simulink model "G2V"  (R2023b)
settings: Solver=VariableStepAuto  StartTime=0.0  StopTime=5  RelTol=1e-3
libraries: spsIGBTDiodeLib x4, spsSeriesRLCBranchLib x3, spsVoltageMeasurementLib x2, spsACVoltageSourceLib x1, spsDiodeLib x1, spsMosfetLib x1, slpidlib x1, spsPWMGeneratorDCDCLib x1, spsTriangleGeneratorLib x1, sps_lib x1
settings Model: Creator=armaan  LastModifiedBy=armaan

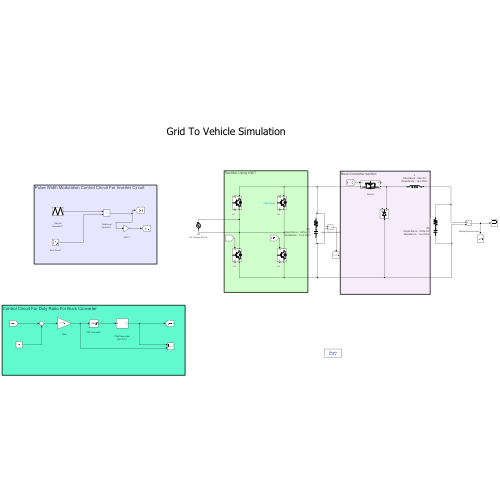
[thumbnail: Simulink's stored preview of the top-level diagram]
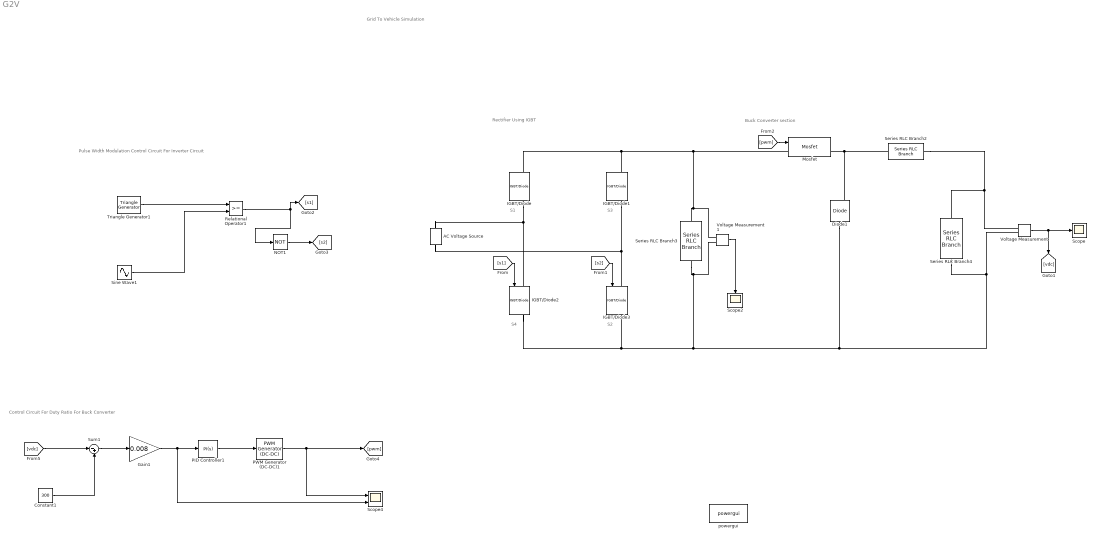
== system G2V ==
  note: Grid To Vehicle Simulation
  note: S1
  note: Buck Converter section
  note: Rectifier Using IGBT
  note: Pulse Width Modulation Control Circuit For Inverter Circuit
  note: Control Circuit For Duty Ratio For Buck Converter
  note: S3
  note: S2
  note: S4
  AC Voltage Source : spsACVoltageSourceLib/AC Voltage Source  Amplitude=440  Phase=0  Frequency=50  SampleTime=0  Measurements=None  BusType=swing  Pref=10e3  Qref=0  Qmin=-inf  Qmax=+inf
      settings: AttributesFormatString=|
      | %<Amplitude>
      | %<Name>
  Constant1 : Constant  Value=300
  Diode1 : spsDiodeLib/Diode  Ron=1e-3  Lon=0  Vf=0  IC=0  UseSnubber=off  Rs=inf  Cs=inf  Measurements=on
  Gain1 : Gain  Gain=0.008
      settings: AttributesFormatString=%<BlockType>
  IGBT/Diode{,1..3} (4 alike) : spsIGBTDiodeLib/IGBT//Diode  Ron=1e-3  Rs=1e5  Cs=inf  Measurements=on
  Mosfet : spsMosfetLib/Mosfet  Ron=0.1  Lon=0  Rd=0.01  Vfd=0  IC=0  Rs=1e5  Cs=inf  Measurements=on
      settings: AttributesFormatString=%<Name>
  NOT1 : Logic  Operator=NOT  IconShape=distinctive  AllPortsSameDT=off  OutDataTypeStr=boolean
      settings: AttributesFormatString=%<Name>
  PID Controller1 : slpidlib/PID Controller  Controller=PI  Form=Parallel  TimeDomain=Continuous-time  UseExternalTs=off  SampleTime=-1  IntegratorMethod=Forward Euler  FilterMethod=Forward Euler  ControllerParametersSource=internal  P=0.1  I=0.1  UseKiTs=off  D=0.1  N=100  UseFilter=on  TunerSelectOption=Transfer Function Based (PID Tuner App)  InitialConditionSource=internal  InitialConditionForIntegrator=0  InitialConditionForFilter=0  DifferentiatorICPrevScaledInput=0  ExternalReset=none  TrackingMode=off  Kt=1  LimitOutput=on  SatLimitsSource=internal  UpperSaturationLimit=1  LowerSaturationLimit=0  LinearizeAsGain=on  AntiWindupMode=none  Kb=1  LimitIntegrator=off  UpperIntegratorSaturationLimit=inf  LowerIntegratorSaturationLimit=-inf  POutMin=[]  POutMax=[]  IOutMin=[]  IOutMax=[]  DOutMin=[]  DOutMax=[]  NOutMin=[]  NOutMax=[]  SumOutMin=[]  SumOutMax=[]  SaturationOutMin=[]  SaturationOutMax=[]  PParamMin=[]  PParamMax=[]  IParamMin=[]  IParamMax=[]  DParamMin=[]  DParamMax=[]  NParamMin=[]  NParamMax=[]  KbParamMin=[]  KbParamMax=[]  KtParamMin=[]  KtParamMax=[]  KbOutMin=[]  KbOutMax=[]  KtOutMin=[]  KtOutMax=[]  IntegratorOutMin=[]  IntegratorOutMax=[]  FilterOutMin=[]  FilterOutMax=[]  SumI1OutMin=[]  SumI1OutMax=[]  SumI2OutMin=[]  SumI2OutMax=[]  SumI3OutMin=[]  SumI3OutMax=[]  SumI4OutMin=[]  SumI4OutMax=[]  SumDOutMin=[]  SumDOutMax=[]  DifferentiatorOutMin=[]  DifferentiatorOutMax=[]  FilterDiffOutCoefMin=[]  FilterDiffOutCoefMax=[]  ReciprocalOutMin=[]  ReciprocalOutMax=[]  SumDenOutMin=[]  SumDenOutMax=[]  SumNumOutMin=[]  SumNumOutMax=[]  DivideOutMin=[]  DivideOutMax=[]  UdiffTsProdOutMin=[]  UdiffTsProdOutMax=[]  NTsProdOutMin=[]  NTsProdOutMax=[]  UintegralTsProdOutMin=[]  UintegralTsProdOutMax=[]  UngainTsProdOutMin=[]  UngainTsProdOutMax=[]  ClampingZeroOutDataTypeStr=Inherit: Inherit via back propagation  ClampingZeroOutMin=[]  ClampingZeroOutMax=[]  FilterDenConstantOutDataTypeStr=Inherit: Inherit via back propagation  FilterDenConstantOutMin=[]  FilterDenConstantOutMax=[]  PCopyOutDataTypeStr=Inherit: Inherit via back propagation  PCopyOutMin=[]  PCopyOutMax=[]  NCopyOutDataTypeStr=Inherit: Inherit via back propagation  NCopyOutMin=[]  NCopyOutMax=[]  IntegratorContinuousStateAttributes=''  IntegratorStateMustResolveToSignalObject=off  IntegratorRTWStateStorageClass=Auto  FilterContinuousStateAttributes=''  FilterStateMustResolveToSignalObject=off  FilterRTWStateStorageClass=Auto  ParallelPVariant=InternalParameters  IdealPVariant=Disabled  IVariant=InternalParameters  DVariant=Disabled  IntegratorVariant=Continuous  SatVariant=Enabled  AWVariant=Passthrough  PCopyVariant=Disabled  TRVariant=Disabled  FdbkBlocksVariant=Forward  IdealPFdbkVariant=Disabled  SatFdbkVariant=Disabled  DerivativeFilterVariant=Disabled  NVariant=Disabled  NCopyVariant=Disabled_SignalSpec  FilterICVariant=Disabled  IntegratorICVariant=InternalICs  ExternalResetVariant=Disabled  TRSumVariant=Passthrough  SumFdbkVariant=Disabled  SumVariant=Sum_PI  TsampFilterVariant=InternalTs  TsampNgainVariant=Passthrough  TsampIntegralVariant=Disabled_SignalSpec  ExternalSaturationOutDataTypeStr=Inherit: Same as second input
      settings: AttributesFormatString=%<Name>
  PWM Generator (DC-DC)1 : spsPWMGeneratorDCDCLib/PWM Generator (DC-DC)  Fsw=15000  Ts=0
      settings: AttributesFormatString=%<Name>
  Relational Operator1 : RelationalOperator  OutDataTypeStr=boolean  RndMeth=Simplest  InputSameDT=off
      settings: AttributesFormatString=%<Name>
  Scope : Scope
  Scope2 : Scope
  Scope4 : Scope  NumInputPorts=2
  Series RLC Branch2 : spsSeriesRLCBranchLib/Series RLC Branch  LConnTagsString=__new0  RConnTagsString=__new0  BranchType=L  Resistance=1e-2  Inductance=30e-3  SetiL0=off  InitialCurrent=0  Capacitance=220e-6  Setx0=off  InitialVoltage=150  Measurements=None
      settings: AttributesFormatString=|
      | %<BranchType>
      | Inductance : %<Inductance> H
      | Resistance : %<Resistance> Ohm
  Series RLC Branch3 : spsSeriesRLCBranchLib/Series RLC Branch  LConnTagsString=__new0  RConnTagsString=__new0  BranchType=RC  Resistance=1e-2  Inductance=200e-6  SetiL0=off  InitialCurrent=0  Capacitance=220e-6  Setx0=off  InitialVoltage=150  Measurements=None
      settings: AttributesFormatString=|
      | %<BranchType>
      | Capacitance : %<Capacitance> F
      | Resistance : %<Resistance> Ohm
  Series RLC Branch4 : spsSeriesRLCBranchLib/Series RLC Branch  LConnTagsString=__new0  RConnTagsString=__new0  BranchType=RC  Resistance=1e-2  Inductance=200e-6  SetiL0=off  InitialCurrent=0  Capacitance=220e-6  Setx0=off  InitialVoltage=150  Measurements=None
      settings: AttributesFormatString=|
      | %<BranchType>
      | Capacitance : %<Capacitance> F
      | Resistance : %<Resistance> Ohm
  Sine Wave1 : Sin  Frequency=100*pi  SampleTime=0
      settings: AttributesFormatString=%<Name>
  Sum1 : Sum  Inputs=|-+
  Triangle Generator1 : spsTriangleGeneratorLib/Triangle Generator  Freq=15000  Phase=0  Ts=0
      settings: AttributesFormatString=%<Name>
  Voltage Measurement : spsVoltageMeasurementLib/Voltage Measurement  PhasorSimulation=off  OutputType=Complex  PSBequivalent=0
      settings: AttributesFormatString=%<Name>
  Voltage Measurement1 : spsVoltageMeasurementLib/Voltage Measurement  PhasorSimulation=off  OutputType=Complex  PSBequivalent=0
      settings: AttributesFormatString=%<Name>
  powergui : sps_lib/powergui  Priority=1  SimulationMode=Discrete  SampleTime=50e-6  frequency=60  Iterations=50  frequencyindice=50  Pbase=100e6  ErrMax=1e-4  UnitsV=kV  UnitsW=MW  buscounter=0  FunctionMessages=off  echomessages=off  EnableUseOfTLC=off  CurrentSourceSwitches=off  DisableSnubberDevices=off  DisableRonSwitches=off  DisableVfSwitches=off  DisplayEquations=off  AutomaticDiscreteSolvers=off  SolverType=Tustin/Backward Euler (TBE)  Interpol=off  ExternalGateDelay=off  methode=off  Ts=100  x0status=blocks  SPID=on  SwTol=0  HookPort=off  NonlinearTolerance=1e-4  nMaxIteration=100  ContinueOnMaxIteration=off  RestoreLinks=warning  ResistiveCurrentMeasurement=off  Frange=[0:2:500]  Ylog=off  Xlog=on  ShowGrid=off  save=off  variable=ZData  structure=0  ZoomFFT=off  StartTime=0.0  cycles=1  DisplayStyle=1  fundamental=60  FreqAxis=off  MaxFrequency=1000  frequencyindicesteady=1  RmsSteady=1  display=off
  wires:
  Voltage Measurement/1 -> [vdc], Scope/1
  [s1] -> IGBT/Diode2/1
  [s2] -> IGBT/Diode3/1
  Relational Operator1/1 -> NOT1/1, [s1]
  NOT1/1 -> [s2]
  Triangle Generator1/1 -> Relational Operator1/1
  Sine Wave1/1 -> Relational Operator1/2
  [pwm] -> Mosfet/1
  Voltage Measurement1/1 -> Scope2/1
  Sum1/1 -> Gain1/1
  PWM Generator (DC-DC)1/1 -> Scope4/1, [pwm]
  Gain1/1 -> Scope4/2, PID Controller1/1
  PID Controller1/1 -> PWM Generator (DC-DC)1/1
  Constant1/1 -> Sum1/2
  [vdc] -> Sum1/1
  connections:
  IGBT/Diode/RConn1 -- AC Voltage Source/RConn1 -- IGBT/Diode2/LConn1
  IGBT/Diode2/RConn1 -- Voltage Measurement1/LConn2 -- Series RLC Branch3/RConn1 -- Diode1/LConn1 -- Voltage Measurement/LConn2 -- Series RLC Branch4/RConn1 -- IGBT/Diode3/RConn1
  Series RLC Branch4/LConn1 -- Series RLC Branch2/LConn1 -- Voltage Measurement/LConn1
  IGBT/Diode1/RConn1 -- AC Voltage Source/LConn1 -- IGBT/Diode3/LConn1
  Diode1/RConn1 -- Series RLC Branch2/RConn1 -- Mosfet/RConn1
  IGBT/Diode1/LConn1 -- Series RLC Branch3/LConn1 -- Voltage Measurement1/LConn1 -- Mosfet/LConn1 -- IGBT/Diode/LConn1
